simulink model "pidLoopTest"  (R2017a)
settings: Solver=VariableStepAuto  StartTime=0.0  StopTime=inf  RelTol=1e-3
values from neighbouring files (symbols this model uses):
  fpgaClk = 50e6    (= 50000000)    [variables.m]
  Ku = 1    [variables.m]
  Tu = 1    [variables.m]
undefined symbols (not defined in the file or in its folder): PWMFreq
libraries: simulink x1
settings Model: Creator=Nicoe Welch  LastModifiedBy=Nicoe Welch

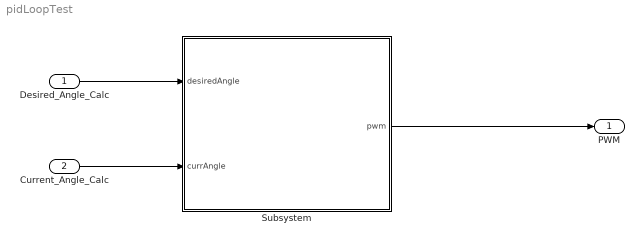
== system pidLoopTest ==
  Desired_Angle_Calc : Inport
  Current_Angle_Calc : Inport  Port=2
  Subsystem : Subsystem
  PWM : Outport
  wires:
  Subsystem/1(pwm) -> PWM/1
  Current_Angle_Calc/1 -> Subsystem/2(currAngle)
  Desired_Angle_Calc/1 -> Subsystem/1(desiredAngle)

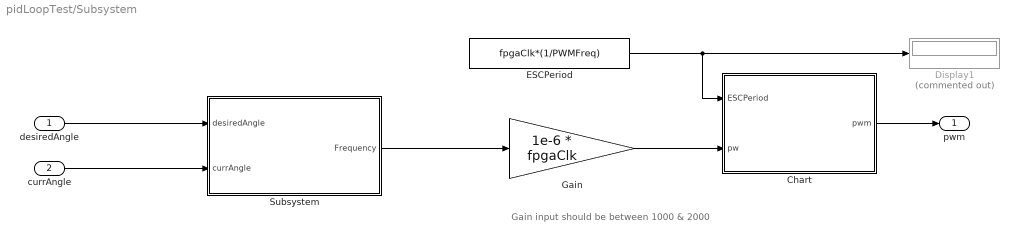
== system pidLoopTest/Subsystem ==
  note: Gain input should be between 1000 & 2000
  desiredAngle : Inport
  currAngle : Inport  Port=2
  Chart : Stateflow chart  TreatAsAtomicUnit=on
  Display1 : Display  Commented=on
  ESCPeriod : Constant  Value=fpgaClk*(1/PWMFreq)  OutDataTypeStr=uint32
  Gain : Gain  Gain=1e-6 * fpgaClk  OutDataTypeStr=Inherit: Same as input
  Subsystem : Subsystem
  pwm : Outport
  wires:
  Gain/1 -> Chart/2(pw)
  ESCPeriod/1 -> Chart/1(ESCPeriod), Display1/1
  Chart/1(pwm) -> pwm/1
  desiredAngle/1 -> Subsystem/1(desiredAngle)
  currAngle/1 -> Subsystem/2(currAngle)
  Subsystem/1(Frequency) -> Gain/1

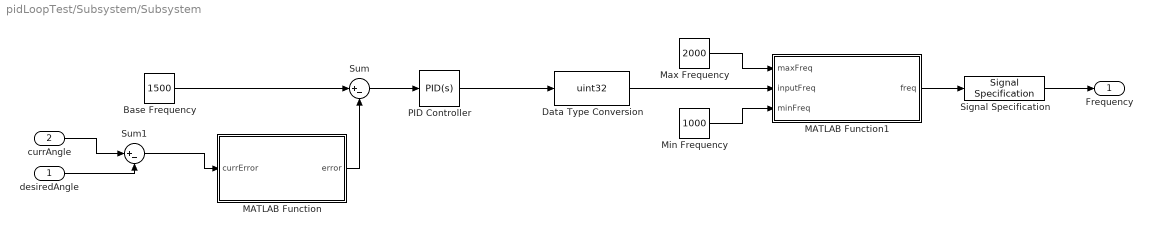
== system pidLoopTest/Subsystem/Subsystem ==
  desiredAngle : Inport
  currAngle : Inport  Port=2
  Base Frequency : Constant  Value=1500
  Data Type Conversion : DataTypeConversion  OutDataTypeStr=uint32
  MATLAB Function : MATLAB Function  TreatAsAtomicUnit=on
  MATLAB Function1 : MATLAB Function  TreatAsAtomicUnit=on
  Max Frequency : Constant  Value=2000  OutDataTypeStr=uint32
  Min Frequency : Constant  Value=1000  OutDataTypeStr=uint32
  PID Controller : simulink/Continuous/PID Controller  Controller=PID  TimeDomain=Continuous-time  SampleTime=-1  IntegratorMethod=Forward Euler  FilterMethod=Forward Euler  Form=Parallel  UseFilter=on  ControllerParametersSource=internal  P=0.6*Ku  I=1.2*Ku/Tu  D=0.6*Ku*Tu/8  N=100  InitialConditionSource=internal  InitialConditionForIntegrator=0  InitialConditionForFilter=0  ExternalReset=none  LimitOutput=off  UpperSaturationLimit=inf  LowerSaturationLimit=-inf  LinearizeAsGain=on  AntiWindupMode=none  Kb=1  TrackingMode=off  Kt=1  PParamMin=[]  PParamMax=[]  IParamMin=[]  IParamMax=[]  DParamMin=[]  DParamMax=[]  NParamMin=[]  NParamMax=[]  KbParamMin=[]  KbParamMax=[]  KtParamMin=[]  KtParamMax=[]  POutMin=[]  POutMax=[]  IOutMin=[]  IOutMax=[]  DOutMin=[]  DOutMax=[]  NOutMin=[]  NOutMax=[]  KbOutMin=[]  KbOutMax=[]  KtOutMin=[]  KtOutMax=[]  IntegratorOutMin=[]  IntegratorOutMax=[]  FilterOutMin=[]  FilterOutMax=[]  SumOutMin=[]  SumOutMax=[]  SumI1OutMin=[]  SumI1OutMax=[]  SumI2OutMin=[]  SumI2OutMax=[]  SumI3OutMin=[]  SumI3OutMax=[]  SumDOutMin=[]  SumDOutMax=[]  SaturationOutMin=[]  SaturationOutMax=[]  IntegratorContinuousStateAttributes=''  IntegratorStateMustResolveToSignalObject=off  IntegratorRTWStateStorageClass=Auto  FilterContinuousStateAttributes=''  FilterStateMustResolveToSignalObject=off  FilterRTWStateStorageClass=Auto  DifferentiatorICPrevScaledInput=0  DifferentiatorOutMin=[]  DifferentiatorOutMax=[]  InitialConditionSetting=State (most efficient)
  Signal Specification : SignalSpecification  OutDataTypeStr=uint32
  Sum : Sum  Inputs=|+-
  Sum1 : Sum  Inputs=|+-
  Frequency : Outport
  wires:
  Sum/1 -> PID Controller/1
  Base Frequency/1 -> Sum/1
  Min Frequency/1 -> MATLAB Function1/3(minFreq)
  Max Frequency/1 -> MATLAB Function1/1(maxFreq)
  desiredAngle/1 -> Sum1/2
  currAngle/1 -> Sum1/1
  MATLAB Function/1(error) -> Sum/2
  Sum1/1 -> MATLAB Function/1(currError)
  MATLAB Function1/1(freq) -> Signal Specification/1
  Signal Specification/1 -> Frequency/1
  PID Controller/1 -> Data Type Conversion/1
  Data Type Conversion/1 -> MATLAB Function1/2(inputFreq)

== stateflow chart pidLoopTest/Subsystem/Chart ==
  settings: executeAtInitialization=1
  state on
    entry: cnt = uint32(0);
    pwm = true;
    during: cnt = cnt + 1;
  state off
    entry: pwm = false;
    during: cnt = cnt + 1;
  (default) -> on
  on -> off : [cnt > pw]
  off -> on : [cnt >= ESCPeriod]
  data: ESCPeriod input uint32; pw input uint32; pwm output boolean; cnt local uint32

== matlab function pidLoopTest/Subsystem/Subsystem/MATLAB Function ==
  data: error output; currError input
function error = fcn(currError)
transError = -.01080*(currError)^3 + .678*(currError)^2 + 2.124*(currError) + 22.653;
if currError < 0
    error = transError * -1;
else
    error = transError;
end

== matlab function pidLoopTest/Subsystem/Subsystem/MATLAB Function1 ==
  data: maxFreq input; inputFreq input; freq output uint32; minFreq input
function freq = fcn(maxFreq,inputFreq, minFreq)
    if( inputFreq > maxFreq ) 
        freq = maxFreq
    elseif ( inputFreq < minFreq ) 
        freq = minFreq
    else 
        freq = inputFreq
    end
